simulink model "MARCH_v1_1"  (R2016a)
settings: Solver=FixedStepDiscrete  StartTime=0.0  StopTime=inf  FixedStep=.001  RelTol=1e-3
PreLoadFcn:
  | load db.mat
  | initialize_model_param
PostLoadFcn:
  | build_location = fullfile(fileparts(which(bdroot)),'build');
  | 
  | set_param(0, 'CacheFolder', build_location);
  | set_param(0, 'CodeGenFolder', build_location);
InitFcn:
  | % Change dir to model location
  | cd(fileparts(which(bdroot)));
  | 
  | % Run init script
  | init_model;
StartFcn:
  | % Make sure we always move back to model folder
  | cd(fileparts(which(bdroot)));
StopFcn:
  | % Make sure we always move back to model folder
  | cd(fileparts(which(bdroot)));
libraries: xpcethercatlib x21, slrtlib x2
CloseFcn:
  | % Make sure we always move back to model folder
  | cd(fileparts(which(bdroot)));
  | 
  | set_param(0, 'CacheFolder', '');
  | set_param(0, 'CodeGenFolder', '');
PauseFcn:
  | % Make sure we always move back to model folder
  | cd(fileparts(which(bdroot)));
ContinueFcn:
  | % Make sure we always move back to model folder
  | cd(fileparts(which(bdroot)));
settings Model: SimulationMode=external  Creator=rtheyyun  LastModifiedBy=Projectmarch
settings SolverCC: EnableConcurrentExecution=on  ConcurrentTasks=on
settings DataIOCC: LimitDataPoints=on  SaveFinalState=on  SaveFormat=StructureWithTime  SignalLoggingSaveFormat=ModelDataLogs  InspectSignalLogs=on
settings OptimizationCC: BlockReduction=off  OptimizeBlockIOStorage=off  BufferReuse=off  GlobalBufferReuse=off  ExpressionFolding=off  ExpressionDepthLimit=2147483647  LocalBlockOutputs=off
settings DebuggingCC: ReadBeforeWriteMsg=DisableAll  WriteAfterWriteMsg=DisableAll  WriteAfterReadMsg=DisableAll  UnderspecifiedInitializationDetection=Classic  MergeDetectMultiDrivingBlocksExec=none  SolverPrmCheckMsg=warning  InheritedTsInSrcMsg=none  FcnCallInpInsideContextMsg=UseLocalSettings  AllowSymbolicDim=off  StateNameClashWarn=warning
settings HardwareCC: ProdBitPerPointer=32  ProdLargestAtomicFloat=None  ProdWordSize=32  ProdLongLongMode=on  ProdHWDeviceType=Generic->32-bit x86 compatible
settings ModelReferenceCC: UpdateModelReferenceTargets=Force  PropagateSignalLabelsOutOfModel=off
settings RTWCC: SystemTargetFile=slrt.tlc  TemplateMakefile=slrt_default_tmf  Description=Simulink Real-Time  RTWVerbose=off  RTWCompilerOptimization=on
settings SimulinkRealTimeCC: GeneratePreprocessorConditionals=Disable all  xPCisModelTimeout=off  xPCModelTimeoutSecs=20  xPCConcurrentTasks=on
settings ConfigComp: CovModelRefEnable=Off  CovSFcnEnable=off
settings ConfigurationSet: Description=SimMechanics 2G

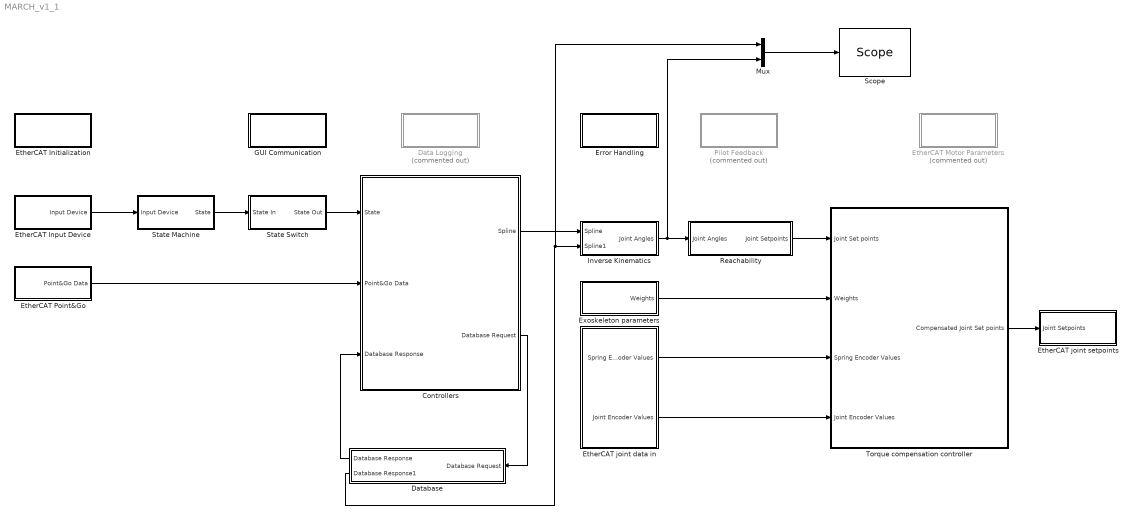
== system MARCH_v1_1 ==
  Controllers : Subsystem
  Data Logging : Subsystem  Commented=on
  Database : Subsystem
  Error Handling : Subsystem
  EtherCAT Initialization : Subsystem
  EtherCAT Input Device : Subsystem
  EtherCAT Motor Parameters : Subsystem  Commented=on
  EtherCAT Point&Go : Subsystem
  EtherCAT joint data in : Subsystem
  EtherCAT joint setpoints : Subsystem
  Exoskeleton parameters : Subsystem
  GUI Communication : Subsystem
  Inverse Kinematics : Subsystem
  Mux : Mux  Inputs=2
  Pilot Feedback : Subsystem  Commented=on
  Reachability : Subsystem
  "Scope " : slrtlib/Displays and Logging/Scope   scopeno=1  scopetype=Target  autostart=on  viewmode=Graphical rolling  formatstr='%15.6f'  grid=on  ylimits=[0,0]  nosamples=25000  noprepostsamples=0  interleave=1  triggermode=FreeRun  triggersignal=1  trigsignalfromport=off  triggerlevel=0.0  triggerslope=Either  triggerscope=1  triggersample=0  filename=data.dat  mode=Lazy  writesize=512  autorestart=off  dynamicfilemode=off  maxwritefilesize=512*1024^2
  State Machine : Subsystem
  State Switch : Subsystem
  Torque compensation controller : Subsystem
  wires:
  Torque compensation controller/1(Compensated Joint Set points) -> EtherCAT joint setpoints/1(Joint Setpoints)
  Reachability/1(Joint Setpoints) -> Torque compensation controller/1(Joint Set points)
  Inverse Kinematics/1(Joint Angles) -> Mux/2, Reachability/1(Joint Angles)
  State Switch/1(State Out) -> Controllers/1(State)
  Controllers/1(Spline) -> Inverse Kinematics/1(Spline)
  State Machine/1(State) -> State Switch/1(State In)
  Controllers/2(Database Request) -> Database/1(Database Request)
  Database/1(Database Response) -> Controllers/3(Database Response)
  EtherCAT joint data in/1(Spring Encoder Values) -> Torque compensation controller/3(Spring Encoder Values)
  EtherCAT joint data in/2(Joint Encoder Values) -> Torque compensation controller/4(Joint Encoder Values)
  Exoskeleton parameters/1(Weights) -> Torque compensation controller/2(Weights)
  EtherCAT Input Device/1(Input Device) -> State Machine/1(Input Device)
  EtherCAT Point&Go/1(Point&Go Data) -> Controllers/2(Point&Go Data)
  Mux/1 -> "Scope "/1
  Database/2(Database Response1) -> Mux/1, Inverse Kinematics/2(Spline1)

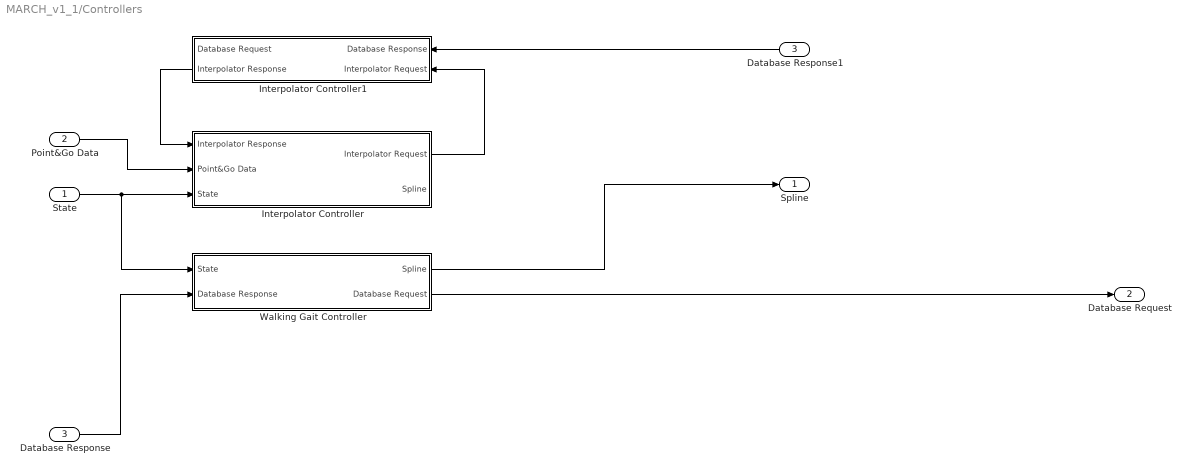
== system MARCH_v1_1/Controllers ==
  State : Inport
  Point&Go Data : Inport  Port=2
  Database Response : Inport  Port=3
  Database Response1 : InportShadow  Port=3
  Interpolator Controller : Subsystem
  Interpolator Controller1 : Subsystem
  Walking Gait Controller : Subsystem
  Spline : Outport
  Database Request : Outport  Port=2
  wires:
  State/1 -> Interpolator Controller/3(State), Walking Gait Controller/1(State)
  Database Response/1 -> Walking Gait Controller/2(Database Response)
  Interpolator Controller/1(Interpolator Request) -> Interpolator Controller1/2(Interpolator Request)
  Interpolator Controller1/2(Interpolator Response) -> Interpolator Controller/1(Interpolator Response)
  Database Response1/1 -> Interpolator Controller1/1(Database Response)
  Walking Gait Controller/2(Database Request) -> Database Request/1
  Walking Gait Controller/1(Spline) -> Spline/1
  Point&Go Data/1 -> Interpolator Controller/2(Point&Go Data)

== system MARCH_v1_1/Data Logging ==

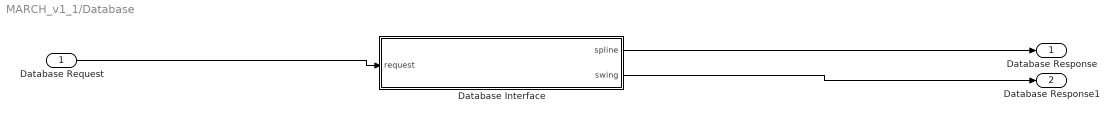
== system MARCH_v1_1/Database ==
  Database Request : Inport
  Database Interface : MATLAB Function  TreatAsAtomicUnit=on
  Database Response : Outport
  Database Response1 : Outport  Port=2
  wires:
  Database Request/1 -> Database Interface/1(request)
  Database Interface/1(spline) -> Database Response/1
  Database Interface/2(swing) -> Database Response1/1

== system MARCH_v1_1/Error Handling ==

== system MARCH_v1_1/EtherCAT Initialization ==
  "EtherCAT Init " : xpcethercatlib/EtherCAT Init   Priority=0  config_file=D:\Software\MATLAB\simulink-models\EtherCAT Config files\quad_slave_both_legs_v1.0.xml  device_id=0  pci_bus=2  pci_slot=0  dctuning=0  enaDebug=off  enaDC=on  errLink=off  masterDbg=off  stateChgDbg=off  baseClock=off  masterCfg=off  logFile='c:\dbglog.txt'  sample_time=0.001000
  Terminator : Terminator
  wires:
  "EtherCAT Init "/1 -> Terminator/1

== system MARCH_v1_1/EtherCAT Input Device ==
  EtherCAT PDO Receive : xpcethercatlib/EtherCAT PDO Receive  Priority=2  sig_name=LHFE.Inputs.jointAngle  sig_offset=208  sig_type=uint32  type_size=32  sig_dim=1  device_id=0  sample_time=0.001000
  Input Device : Outport
  wires:
  EtherCAT PDO Receive/1 -> Input Device/1

== system MARCH_v1_1/EtherCAT Motor Parameters ==

== system MARCH_v1_1/EtherCAT Point&Go ==
  EtherCAT PDO Receive : xpcethercatlib/EtherCAT PDO Receive  Priority=2  sig_name=LHFE.Inputs.jointAngle  sig_offset=208  sig_type=uint32  type_size=32  sig_dim=1  device_id=0  sample_time=0.001000
  Point&Go Data : Outport
  wires:
  EtherCAT PDO Receive/1 -> Point&Go Data/1

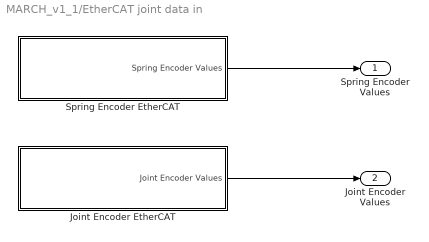
== system MARCH_v1_1/EtherCAT joint data in ==
  Joint Encoder EtherCAT : Subsystem
  Spring Encoder EtherCAT : Subsystem
  Spring Encoder Values : Outport
  Joint Encoder Values : Outport  Port=2
  wires:
  Spring Encoder EtherCAT/1(Spring Encoder Values) -> Spring Encoder Values/1
  Joint Encoder EtherCAT/1(Joint Encoder Values) -> Joint Encoder Values/1

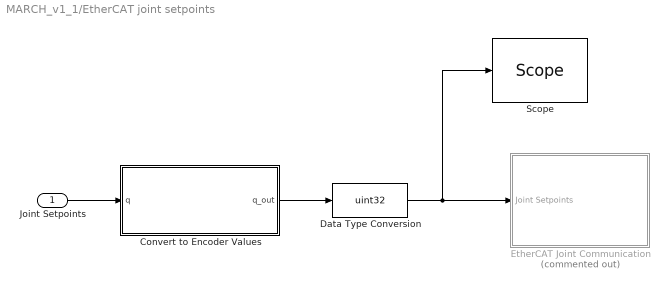
== system MARCH_v1_1/EtherCAT joint setpoints ==
  Joint Setpoints : Inport
  Convert to Encoder Values : MATLAB Function  TreatAsAtomicUnit=on
  Data Type Conversion : DataTypeConversion  OutDataTypeStr=uint32
  EtherCAT Joint Communication : Subsystem  Commented=on
  "Scope " : slrtlib/Displays and Logging/Scope   scopeno=2  scopetype=Target  autostart=on  viewmode=Graphical rolling  formatstr='%15.6f'  grid=on  ylimits=[0,0]  nosamples=25000  noprepostsamples=3  interleave=1  triggermode=FreeRun  triggersignal=1  trigsignalfromport=off  triggerlevel=0.0  triggerslope=Either  triggerscope=1  triggersample=0  filename=data.dat  mode=Lazy  writesize=512  autorestart=off  dynamicfilemode=off  maxwritefilesize=512*1024^2
  wires:
  Convert to Encoder Values/1(q_out) -> Data Type Conversion/1
  Joint Setpoints/1 -> Convert to Encoder Values/1(q)
  Data Type Conversion/1 -> "Scope "/1, EtherCAT Joint Communication/1(Joint Setpoints)

== system MARCH_v1_1/Exoskeleton parameters ==
  Weights : Outport

== system MARCH_v1_1/GUI Communication ==

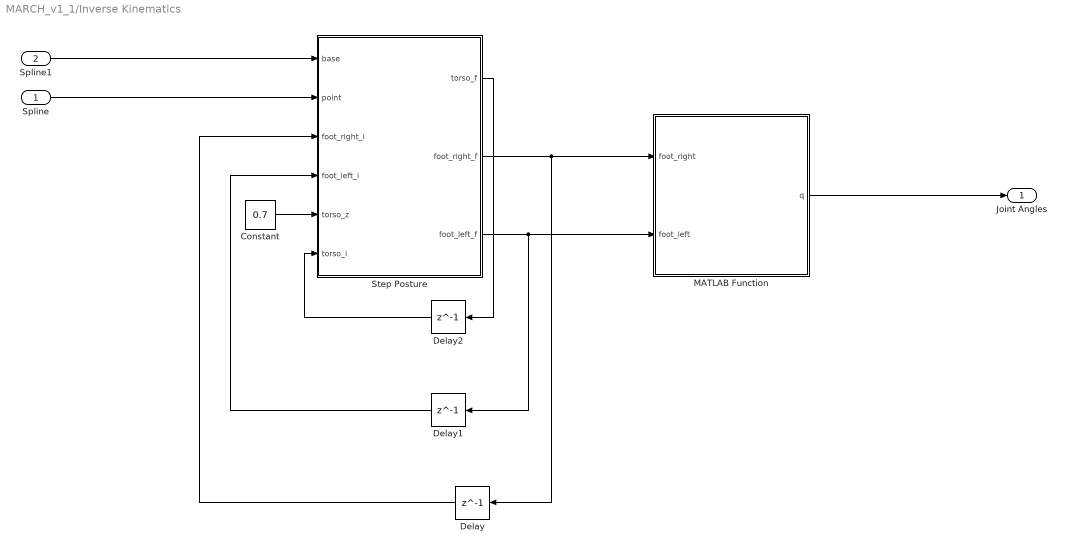
== system MARCH_v1_1/Inverse Kinematics ==
  Spline : Inport
  Spline1 : Inport  Port=2
  Constant : Constant  Value=0.7
  Delay : Delay  DelayLength=1
  Delay1 : Delay  DelayLength=1
  Delay2 : Delay  DelayLength=1
  MATLAB Function : MATLAB Function  TreatAsAtomicUnit=on
  Step Posture : MATLAB Function  TreatAsAtomicUnit=on
  Joint Angles : Outport
  wires:
  MATLAB Function/1(q) -> Joint Angles/1
  Step Posture/2(foot_right_f) -> Delay/1, MATLAB Function/1(foot_right)
  Step Posture/3(foot_left_f) -> Delay1/1, MATLAB Function/2(foot_left)
  Spline/1 -> Step Posture/2(point)
  Delay/1 -> Step Posture/3(foot_right_i)
  Delay1/1 -> Step Posture/4(foot_left_i)
  Constant/1 -> Step Posture/5(torso_z)
  Step Posture/1(torso_f) -> Delay2/1
  Delay2/1 -> Step Posture/6(torso_i)
  Spline1/1 -> Step Posture/1(base)

== system MARCH_v1_1/Pilot Feedback ==

== system MARCH_v1_1/Reachability ==
  Joint Angles : Inport
  MATLAB Function : MATLAB Function  TreatAsAtomicUnit=on
  Joint Setpoints : Outport
  wires:
  Joint Angles/1 -> MATLAB Function/1(q)
  MATLAB Function/1(q_out) -> Joint Setpoints/1

== system MARCH_v1_1/State Machine ==
  Input Device : Inport
  Constant : Constant  Value=2
  State : Outport
  wires:
  Constant/1 -> State/1

== system MARCH_v1_1/State Switch ==
  State In : Inport
  State Out : Outport
  wires:
  State In/1 -> State Out/1

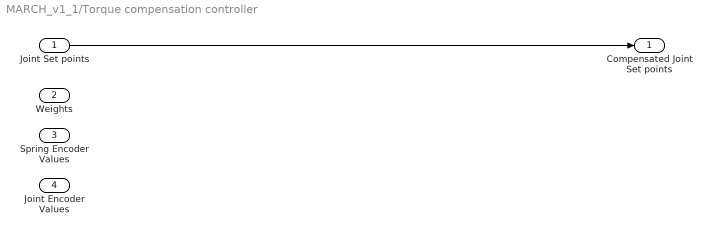
== system MARCH_v1_1/Torque compensation controller ==
  Joint Set points : Inport
  Weights : Inport  Port=2
  Spring Encoder Values : Inport  Port=3
  Joint Encoder Values : Inport  Port=4
  Compensated Joint Set points : Outport
  wires:
  Joint Set points/1 -> Compensated Joint Set points/1

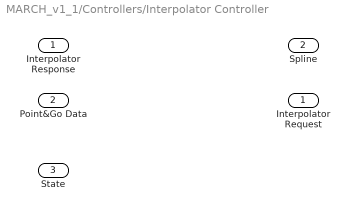
== system MARCH_v1_1/Controllers/Interpolator Controller ==
  Interpolator Response : Inport
  Point&Go Data : Inport  Port=2
  State : Inport  Port=3
  Interpolator Request : Outport
  Spline : Outport  Port=2

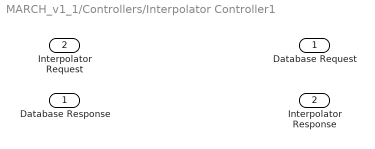
== system MARCH_v1_1/Controllers/Interpolator Controller1 ==
  Database Response : Inport
  Interpolator Request : Inport  Port=2
  Database Request : Outport
  Interpolator Response : Outport  Port=2

== system MARCH_v1_1/Controllers/Walking Gait Controller ==
  State : Inport
  Database Response : Inport  Port=2
  Spline : Outport
  Database Request : Outport  Port=2
  wires:
  State/1 -> Database Request/1
  Database Response/1 -> Spline/1

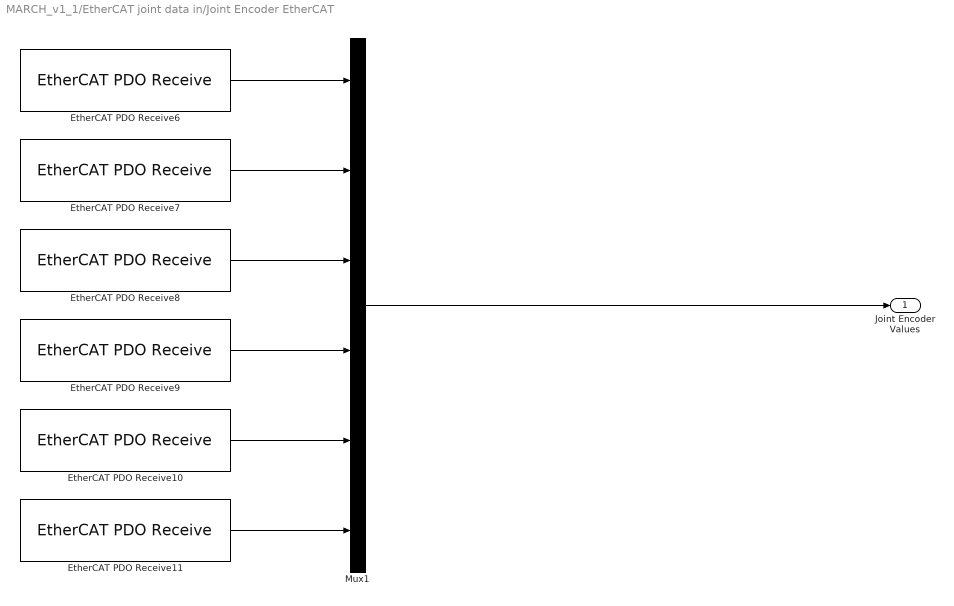
== system MARCH_v1_1/EtherCAT joint data in/Joint Encoder EtherCAT ==
  EtherCAT PDO Receive{6..11} (6 alike) : xpcethercatlib/EtherCAT PDO Receive  Priority=2  sig_name=LHFE.Inputs.jointAngle  sig_offset=208  sig_type=uint32  type_size=32  sig_dim=1  device_id=0  sample_time=0.001000
  Mux1 : Mux  Inputs=6
  Joint Encoder Values : Outport
  wires:
  EtherCAT PDO Receive8/1 -> Mux1/3
  EtherCAT PDO Receive9/1 -> Mux1/4
  EtherCAT PDO Receive7/1 -> Mux1/2
  EtherCAT PDO Receive6/1 -> Mux1/1
  EtherCAT PDO Receive10/1 -> Mux1/5
  EtherCAT PDO Receive11/1 -> Mux1/6
  Mux1/1 -> Joint Encoder Values/1

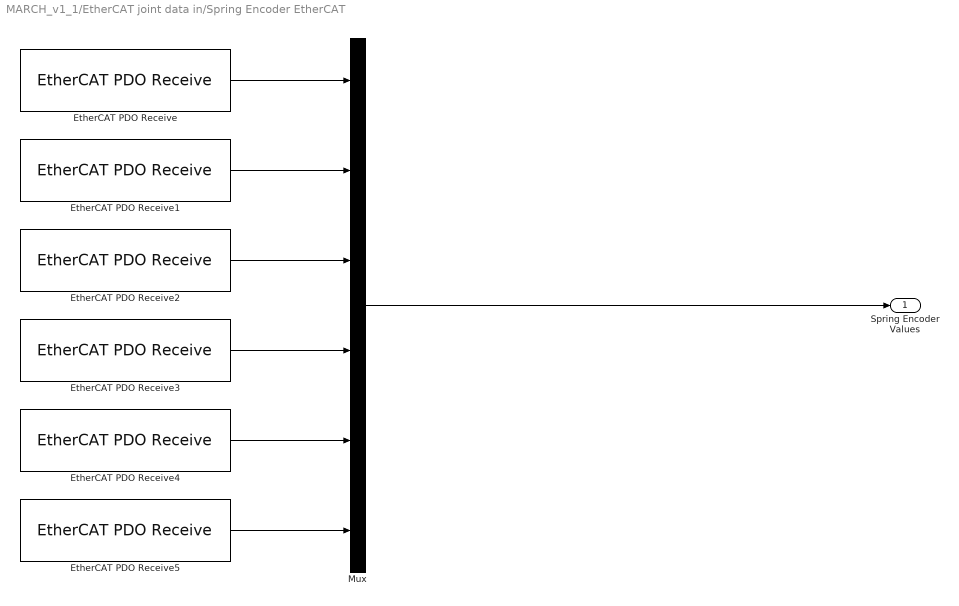
== system MARCH_v1_1/EtherCAT joint data in/Spring Encoder EtherCAT ==
  EtherCAT PDO Receive{,1..5} (6 alike) : xpcethercatlib/EtherCAT PDO Receive  Priority=2  sig_name=LHFE.Inputs.jointAngle  sig_offset=208  sig_type=uint32  type_size=32  sig_dim=1  device_id=0  sample_time=0.001000
  Mux : Mux  Inputs=6
  Spring Encoder Values : Outport
  wires:
  EtherCAT PDO Receive2/1 -> Mux/3
  EtherCAT PDO Receive4/1 -> Mux/5
  Mux/1 -> Spring Encoder Values/1
  EtherCAT PDO Receive5/1 -> Mux/6
  EtherCAT PDO Receive1/1 -> Mux/2
  EtherCAT PDO Receive/1 -> Mux/1
  EtherCAT PDO Receive3/1 -> Mux/4

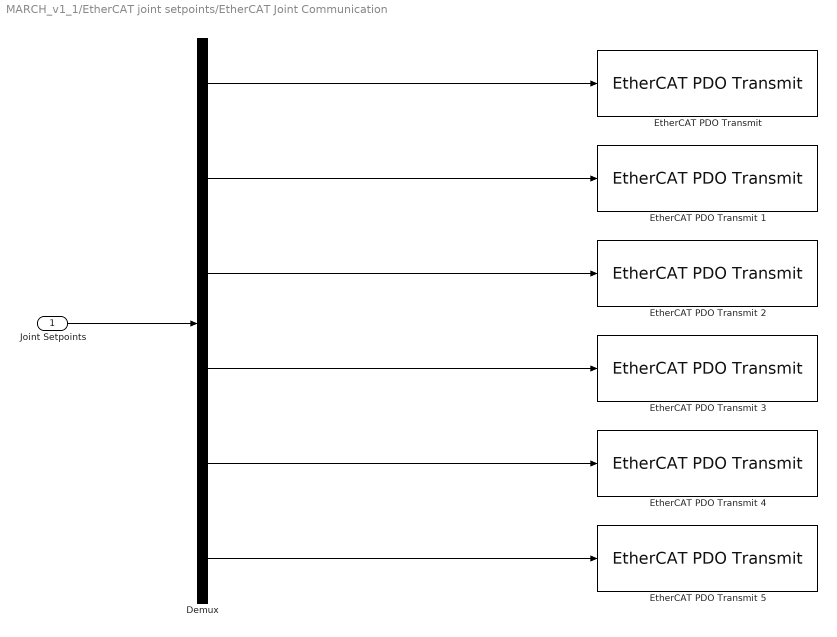
== system MARCH_v1_1/EtherCAT joint setpoints/EtherCAT Joint Communication ==
  Joint Setpoints : Inport
  Demux : Demux  Outputs=6
  "EtherCAT PDO Transmit " : xpcethercatlib/EtherCAT PDO Transmit   Priority=3  sig_name=LKFE.Outputs.jointSetpoint  sig_offset=496  sig_type=uint32  type_size=32  sig_dim=1  device_id=0  sample_time=0.001000
  EtherCAT PDO Transmit 1 : xpcethercatlib/EtherCAT PDO Transmit   Priority=3  sig_name=LHFE.Outputs.data0  sig_offset=240  sig_type=uint32  type_size=32  sig_dim=1  device_id=0  sample_time=0.001000
  EtherCAT PDO Transmit 2 : xpcethercatlib/EtherCAT PDO Transmit   Priority=3  sig_name=LHFE.Outputs.data0  sig_offset=240  sig_type=uint32  type_size=32  sig_dim=1  device_id=0  sample_time=0.001000
  EtherCAT PDO Transmit 3 : xpcethercatlib/EtherCAT PDO Transmit   Priority=3  sig_name=LHFE.Outputs.data0  sig_offset=240  sig_type=uint32  type_size=32  sig_dim=1  device_id=0  sample_time=0.001000
  EtherCAT PDO Transmit 4 : xpcethercatlib/EtherCAT PDO Transmit   Priority=3  sig_name=RHFE.Outputs.jointSetpoint  sig_offset=12496  sig_type=uint32  type_size=32  sig_dim=1  device_id=0  sample_time=0.001000
  EtherCAT PDO Transmit 5 : xpcethercatlib/EtherCAT PDO Transmit   Priority=3  sig_name=RKFE.Outputs.jointSetpoint  sig_offset=12784  sig_type=uint32  type_size=32  sig_dim=1  device_id=0  sample_time=0.001000
  wires:
  Demux/5 -> EtherCAT PDO Transmit 4/1
  Demux/6 -> EtherCAT PDO Transmit 5/1
  Demux/4 -> EtherCAT PDO Transmit 3/1
  Demux/1 -> "EtherCAT PDO Transmit "/1
  Demux/3 -> EtherCAT PDO Transmit 2/1
  Demux/2 -> EtherCAT PDO Transmit 1/1
  Joint Setpoints/1 -> Demux/1

== matlab function MARCH_v1_1/Reachability/MATLAB Function ==
  data: q input; q_out output; err output
function [q_out, err] = fcn(q)

joint_limit_min = [-20 -109 -3 -23 -109 -3]/180*pi;
joint_limit_max = [23 21 121 20 21 121]/180*pi;

n = size(q,1);
%% Check if all joints are within limits

err = imag(q)~=0 | q<repmat(joint_limit_min,n,1) | q>repmat(joint_limit_max,n,1);
q_out = q;

== matlab function MARCH_v1_1/Inverse Kinematics/MATLAB Function ==
  data: foot_right input; q output; foot_left input; par parameter
function q = fcn(foot_right, foot_left, par)

q = inverse_kinematics(foot_right, foot_left, par);

== matlab function MARCH_v1_1/Database/Database Interface ==
  data: request input; spline output; s parameter; swing output
function [spline,swing] = databaseInterface(request, s)
%#codegen
persistent i req base


if(isempty(i))
   i = zeros(1); 
end

if(isempty(req))
   req = zeros(1); 
end

if(isempty(base))
   base = zeros(1); 
end

if (req ~= request)
    req = request;
    i = 0;
end

if i < length(s(1).spline)
    i = i+1;
else 
    i = 0;
    if base == 0
        base = 1;
    else 
        base = 0;
    end
end

spline = s(req).spline(:,i);
swing = base;

== matlab function MARCH_v1_1/Inverse Kinematics/Step Posture ==
  data: base input; torso_f output; point input; foot_right_f output; foot_right_i input; foot_left_i input; torso_z input; foot_left_f output; par parameter; torso_i input
function [torso_f,foot_right_f,foot_left_f] = step_posture(base,point,foot_right_i,foot_left_i, torso_z, par, torso_i)
%% Initialize parameters
point = point';
n = size(point,1);

%% Compute the final x and y positions of torso and feet
if base == 1 %left swing leg
    torso_d = (point+foot_right_i)/2-repmat([par.pelvis_depth 0 0],n,1); %keep torso inbetween stance and swing foot
    foot_right_f = foot_right_i-torso_d; %final right foot position with respect to torso
    foot_left_f = point-torso_d; %final left foot position with respect to torso
else %right swing leg
    torso_d = (point+foot_left_i)/2-repmat([par.pelvis_depth 0 0],n,1); %keep torso inbetween stance and swing foot
    foot_left_f = foot_left_i-torso_d; %final left foot position with respect to torso
    foot_right_f = point-torso_d; %final right foot position with respect to torso
end
torso_f = torso_i+torso_d; %final torso position with respect to world

%% Compute final z positions of torso and feet
% torso height is adapted to keep the stance leg fully stretched
if base == 1 %left swing leg
    torso_f(:,3) = sqrt(torso_z^2+par.pelvis_width^2-(torso_f(:,1)+par.pelvis_depth-torso_i(:,1)-foot_right_i(:,1)).^2-(torso_f(:,2)-par.torso_width-torso_i(:,2)-foot_right_i(:,2)).^2);
else %right swing leg
    torso_f(:,3) = sqrt(torso_z^2+par.pelvis_width^2-(torso_f(:,1)+par.pelvis_depth-torso_i(:,1)-foot_left_i(:,1)).^2-(torso_f(:,2)+par.torso_width-torso_i(:,2)-foot_left_i(:,2)).^2);
end

foot_right_f(:,3) = -torso_f(:,3);
foot_left_f(:,3) = -torso_f(:,3);

== matlab function MARCH_v1_1/EtherCAT joint setpoints/Convert to Encoder Values ==
  data: q input; q_out output
function q_out = convertToEncoderValues(q)

% RHAA
% RHFE
% RKFE
% LHAA
% LHFE
% LKFE

RHAA_scale = (391444-360746)/(128/180*pi);
RHAA_offset = RHAA_scale * (18/180*pi) + 340338;

RHFE_scale = (435150-340338)/(128/180*pi);
RHFE_offset = RHFE_scale * (18/180*pi) + 340338;

RKFE_scale = (393895-305130)/(121.5/180*pi);
RKFE_offset = RKFE_scale * (120/180*pi) + 305130;

LHAA_scale = (435150-340338)/(128/180*pi);
LHAA_offset = LHAA_scale * (18/180*pi) + 340338;

LHFE_scale = (490459-396620)/(128/180*pi);
LHFE_offset = LHFE_scale * (18/180*pi) + 490469;

LKFE_scale = (460672-371304)/(121.5/180*pi);
LKFE_offset = LKFE_scale * (120/180*pi) + 460672;

% convert joint angles to encoder values
q_out = [q(1)*RHAA_scale + RHAA_offset;
         q(2)*RHFE_scale + RHFE_offset;
         q(3)*RKFE_scale + RKFE_offset;
         q(4)*LHAA_scale + LHAA_offset;
         q(5)*LHFE_scale + LHFE_offset;
         q(6)*LKFE_scale + LKFE_offset];
